simulink model "ASM1_Influentmodelprimary"  (Simulink 8.0)
settings: Solver=ode15s  SolverMode=SingleTasking  StartTime=0.0  StopTime=728  FixedStep=0.01  RelTol=1e-5  AbsTol=1e-8
values from neighbouring files (symbols this model uses):
  ASM1_PARS = [ mu_H  K_S  K_OH  K_NO  b_H  mu_A  K_NH  K_OA  b_A  ny_g  k_a  k_h  K_X  ny_h  Y_H  Y_A  f_P  i_XB  i_XP X_I2TSS  X_S2TSS  X_BH2TSS  X_BA2TSS  X_P2TSS ]    [ASM1_Influent_init.m]    (also in ASM1_Influent_init_MC_IBU.m; ASM1_Influent_init_MC_T.m; ASM1_Influent_init_MC_TSS.m; ASM1_Influent_init_dry.m)
  PAR_P = [ f_corr  f_X  t_m  f_PS ]    [ASM1_Influent_init.m]    (also in ASM1_Influent_init_dry.m; ASM1_Influent_init_dry_cal.m; ASM1_Influent_init_dry_cal2.m)
  TEMPMODEL = [ 1 ]    [ASM1_Influent_init.m]    (also in ASM1_Influent_init_dry.m; ASM1_Influent_init_dry_cal.m; ASM1_Influent_init_dry_cal2.m)
  VOL_P = 900    [ASM1_Influent_init.m]    (also in ASM1_Influent_init_dry.m; ASM1_Influent_init_dry_cal.m; ASM1_Influent_init_dry_cal2.m)
  XINIT_P = [ S_I_P  S_S_P  X_I_P  X_S_P  X_BH_P  X_BA_P  X_P_P  S_O_P  S_NO_P  S_NH_P  S_ND_P  X_ND_P  S_ALK_P TSS_P Q_P T_P S_D1_P S_D2_P S_D3_P X_D4_P X_D5_P ]    [ASM1_Influent_init.m]    (also in ASM1_Influent_init_dry.m; ASM1_Influent_init_dry_cal.m; ASM1_Influent_init_dry_cal2.m)
  XVEKTOR_P = [0  0  1  1  1  1  1  0  0  0  0  1  0  0  0  0  0  0  0  1  1]    [ASM1_Influent_init.m]    (also in ASM1_Influent_init_dry.m; ASM1_Influent_init_dry_cal.m; ASM1_Influent_init_dry_cal2.m)
settings Model: Creator=ielulf  LastModifiedBy=lasn  ExtModeTrigMode=oneshot  ExtModeArmWhenConnect=off  ExtModeAutoUpdateStatusClock=off  BufferReuse=off
settings DataIOCC: InitialState=xFinal  LimitDataPoints=off  SignalLoggingSaveFormat=ModelDataLogs  SaveOutput=off  TimeSaveName=t  SignalLoggingName=sigsOut  OutputOption=SpecifiedOutputTimes  OutputTimes=[0:(1/96):609]
settings OptimizationCC: BlockReduction=off  BooleanDataType=off  InlineInvariantSignals=on  OptimizeBlockIOStorage=off  BufferReuse=off  ExpressionFolding=off  LocalBlockOutputs=off  InitFltsAndDblsToZero=on
settings DebuggingCC: SaveWithParameterizedLinksMsg=none  SignalResolutionControl=TryResolveAllWithWarning  SolverPrmCheckMsg=none  InheritedTsInSrcMsg=none  MultiTaskDSMMsg=warning  MultiTaskCondExecSysMsg=none  FcnCallInpInsideContextMsg=UseLocalSettings  UnconnectedOutputMsg=none  StrictBusMsg=None
settings HardwareCC: TargetUnknown=on
settings RTWCC: TemplateMakefile=grt_unix.tmf  IncludeERTFirstTime=on
settings GRTTargetCC: TargetFcnLib=ansi_tfl_tmw.mat  CombineOutputUpdateFcns=off  GRTInterface=on

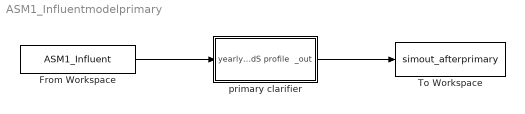
== system ASM1_Influentmodelprimary ==
  From Workspace : FromWorkspace  VariableName=ASM1_Influent  SampleTime=0
  To Workspace : ToWorkspace  VariableName=simout_afterprimary  SampleTime=-1
  primary clarifier : Subsystem
  wires:
  primary clarifier/1(_out) -> To Workspace/1
  From Workspace/1 -> primary clarifier/1(yearly_indS profile)

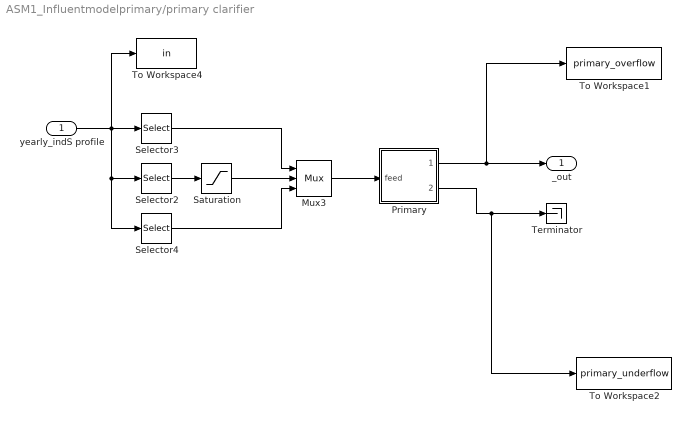
== system ASM1_Influentmodelprimary/primary clarifier ==
  yearly_indS profile : Inport
  Mux3 : Mux  Inputs=3
  Primary : Subsystem
  Saturation : Saturate  UpperLimit=60000  LowerLimit=0
  Selector2 : Selector  InputPortWidth=21  IndexOptions=Index vector (dialog)  Indices=[15]  OutputSizes=1
  Selector3 : Selector  InputPortWidth=21  IndexOptions=Index vector (dialog)  Indices=[1:14]  OutputSizes=1
  Selector4 : Selector  InputPortWidth=21  IndexOptions=Index vector (dialog)  Indices=[16:21]  OutputSizes=1
  Terminator : Terminator
  To Workspace1 : ToWorkspace  VariableName=primary_overflow
  To Workspace2 : ToWorkspace  VariableName=primary_underflow
  To Workspace4 : ToWorkspace  VariableName=in
  _out : Outport
  wires:
  yearly_indS profile/1 -> To Workspace4/1, Selector3/1, Selector2/1, Selector4/1
  Primary/1(o_flow) -> _out/1, To Workspace1/1
  Primary/2(u_flow) -> Terminator/1, To Workspace2/1
  Selector2/1 -> Saturation/1
  Saturation/1 -> Mux3/2
  Selector3/1 -> Mux3/1
  Selector4/1 -> Mux3/3
  Mux3/1 -> Primary/1(feed)

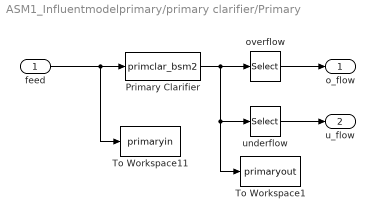
== system ASM1_Influentmodelprimary/primary clarifier/Primary ==
  feed : Inport
  Primary Clarifier : S-Function  FunctionName=primclar_bsm2  Parameters=XINIT_P,XVEKTOR_P,PAR_P,VOL_P,ASM1_PARS,TEMPMODEL  EnableBusSupport=off
  To Workspace1 : ToWorkspace  VariableName=primaryout
  To Workspace11 : ToWorkspace  VariableName=primaryin
  overflow : Selector  InputPortWidth=63  IndexOptions=Index vector (dialog)  Indices=[1:21]  OutputSizes=1
  underflow : Selector  InputPortWidth=63  IndexOptions=Index vector (dialog)  Indices=[22:42]  OutputSizes=1
  o_flow : Outport
  u_flow : Outport  Port=2
  wires:
  Primary Clarifier/1 -> To Workspace1/1, underflow/1, overflow/1
  feed/1 -> Primary Clarifier/1, To Workspace11/1
  underflow/1 -> u_flow/1
  overflow/1 -> o_flow/1
